simulink subsystem "Plant_and_Environment_Model"  (R2020a)
settings: Solver=VariableStepAuto  StartTime=0.0  StopTime=10.0  RelTol=1e-3
values from neighbouring files (symbols this model uses):
  a_rad = deg2rad(a)    [plant_init.m]
  AF = [0.12, 0.22, 0.292]    [plant_init.m]
  l1 = [ sin(a14),-cos(a14), 0,         (D14(3)-RG(3)+PZ(1)*dz)*cos(a14),         (D14(3)-RG(3)+PZ(1)*dz)*sin(a14),         -hypot( D14(1)-RG(1), D14(2)-RG(2))]    [GetAuvSimAndJacobian.m]    (also in plant_init.m = [(D14(3)-RB(3)+PZ(1)*dz),     (D14(3)-RB(3)+PZ(1)*dz),     -)
  l2 = [ sin(a14), cos(a14), 0,          -(D14(3)-RG(3)+PZ(2)*dz)*cos(a14),          (D14(3)-RG(3)+PZ(2)*dz)*sin(a14),          -hypot( D14(1)+RG(1), D14(2)-RG(2))]    [GetAuvSimAndJacobian.m]    (also in plant_init.m = [-(D14(3)-RB(3)+PZ(2)*dz),      (D14(3)-RB(3)+PZ(2)*dz),    )
  l3 = [ sin(a14),-cos(a14), 0,         (D14(3)-RG(3)+PZ(3)*dz)*cos(a14),          (D14(3)-RG(3)+PZ(3)*dz)*sin(a14),          hypot(D14(1)+RG(1), D14(2)+RG(2))]    [GetAuvSimAndJacobian.m]    (also in plant_init.m = [(D14(3)-RB(3)+PZ(3)*dz),      (D14(3)-RB(3)+PZ(3)*dz),     )
  l4 = [ sin(a14), cos(a14), 0,         -(D14(3)-RG(3)+PZ(4)*dz)*cos(a14),          (D14(3)-RG(3)+PZ(4)*dz)*sin(a14),          hypot(D14(1)-RG(1), D14(2)+RG(2))]    [GetAuvSimAndJacobian.m]    (also in plant_init.m = [-(D14(3)-RB(3)+PZ(4)*dz),      (D14(3)-RB(3)+PZ(4)*dz),    )
  l5 = [0, 0, 1, (D58(2)-RG(2)+PZ(1)*dz),          -(D58(1)-RG(1)+PZ(1)*dz), 0]    [GetAuvSimAndJacobian.m]    (also in plant_init.m = [(D58(2)-RB(2)+PZ(1)*dz),      -(D58(1)-RB(1)+PZ(1)*dz), 0])
  l6 = [0, 0,-1,-(D58(2)-RG(2)+PZ(2)*dz),           -(D58(1)+RG(1)+PZ(2)*dz), 0]    [GetAuvSimAndJacobian.m]    (also in plant_init.m = [-(D58(2)-RB(2)+PZ(2)*dz),       -(D58(1)+RB(1)+PZ(2)*dz), 0)
  l7 = [0, 0, 1,-(D58(2)+RG(2)+PZ(3)*dz),         (D58(1)+RG(1)+PZ(3)*dz), 0]    [GetAuvSimAndJacobian.m]    (also in plant_init.m = [-(D58(2)+RB(2)+PZ(3)*dz),     (D58(1)+RB(1)+PZ(3)*dz), 0])
  l8 = [0, 0,-1, (D58(2)+RG(2)+PZ(4)*dz),          (D58(1)-RG(1)+PZ(2)*dz), 0]    [GetAuvSimAndJacobian.m]    (also in plant_init.m = [(D58(2)+RB(2)+PZ(4)*dz),      (D58(1)-RB(1)+PZ(2)*dz), 0])
  mass = cf.mass    [main_adaptive_mpc.m]    (also in plant_init.m = 33.95)
  N = [-39.9215617836 -39.7361560536 -39.4691718024 -38.8907059248 -38.267742672 -37.9562610456 -37.5112872936 -37.2888004176 -36.7993292904 -36.4433502888 -35.8648844112 -35.1974237832 ... (201 elements, 201x1)]    [matlab.mat]    (also in plant_init.m = T200Spec16V{:,6})
  PWM = [1100 1104 1108 1112 1116 1120 1124 1128 1132 1136 1140 1144 ... (201 elements, 201x1)]    [matlab.mat]    (also in plant_init.m = T200Spec16V{:,1})
  RB = [ 0.001,      -0.003,       0.027]    [plant_init.m]
  RG = [ 0.001,      -0.003,       0.027]    [plant_init.m]
  rho = 998    [plant_init.m]
  volume = 0.027    [plant_init.m]
libraries: sharedtransform x11, vrlib x9, shared6dof x1, aerolibasang x1
(part 2 of 2)

== system Plant_and_Environment_Model/Propulsion Forces & Moments/Force and moments due to Thrust/Thrust to Propulsion /Moment computation/Moment Moteur 4 ==
  Thrust : Inport
  Constant : Constant  Value=[a;b;c]
  Cross Product : vrlib/Utilities/Cross Product
  Moment : Outport  VectorParamsAs1DForOutWhenUnconnected=off
  wires:
  Cross Product/1 -> Moment/1
  Thrust/1 -> Cross Product/2
  Constant/1 -> Cross Product/1

== system Plant_and_Environment_Model/Propulsion Forces & Moments/Force and moments due to Thrust/Thrust to Propulsion /Moment computation/Moment Moteur 5 ==
  Thrust : Inport
  Constant : Constant  Value=[a;b;c]
  Cross Product : vrlib/Utilities/Cross Product
  Moment : Outport  VectorParamsAs1DForOutWhenUnconnected=off
  wires:
  Constant/1 -> Cross Product/1
  Thrust/1 -> Cross Product/2
  Cross Product/1 -> Moment/1

== system Plant_and_Environment_Model/Propulsion Forces & Moments/Force and moments due to Thrust/Thrust to Propulsion /Moment computation/Moment Moteur 6 ==
  Thrust : Inport
  Constant : Constant  Value=[a;b;c]
  Cross Product : vrlib/Utilities/Cross Product
  Moment : Outport  VectorParamsAs1DForOutWhenUnconnected=off
  wires:
  Constant/1 -> Cross Product/1
  Thrust/1 -> Cross Product/2
  Cross Product/1 -> Moment/1

== system Plant_and_Environment_Model/Propulsion Forces & Moments/Force and moments due to Thrust/Thrust to Propulsion /Moment computation/Moment Moteur 7 ==
  Thrust : Inport
  Constant : Constant  Value=[a;b;c]
  Cross Product : vrlib/Utilities/Cross Product
  Moment : Outport  VectorParamsAs1DForOutWhenUnconnected=off
  wires:
  Constant/1 -> Cross Product/1
  Thrust/1 -> Cross Product/2
  Cross Product/1 -> Moment/1

== system Plant_and_Environment_Model/Propulsion Forces & Moments/Force and moments due to Thrust/Thrust to Propulsion /Moment computation/Moment Moteur 8 ==
  Thrust : Inport
  Constant : Constant  Value=[a;b;c]
  Cross Product : vrlib/Utilities/Cross Product
  Moment : Outport  VectorParamsAs1DForOutWhenUnconnected=off
  wires:
  Constant/1 -> Cross Product/1
  Thrust/1 -> Cross Product/2
  Cross Product/1 -> Moment/1

== matlab function Plant_and_Environment_Model/Environmental Forces & Moments/Hydrodynamic Forces/Hydrodynamic Forces - Accurate/Force Exerted due to Lift (Body Axis)/MATLAB Function ==
  data: u input; y output
function y = fcn(u)
if u>pi/2
    u = u-pi;
elseif u < -pi/2
    u = u + pi;
end

y = 1 * (u) + 0;

== matlab function Plant_and_Environment_Model/Propulsion Forces & Moments/Input commands to Thrust/PWM Signals to Thrust /MATLAB Function ==
  data: u input; y output
function y = Normalize(u)
y = (u-1500)*150/400;

== matlab function Plant_and_Environment_Model/Propulsion Forces & Moments/Input commands to Thrust/PWM Signals to Thrust /MATLAB Function1 ==
  data: u input; y output
function y = Normalize(u)
y = (u-1500)*150/400;

== matlab function Plant_and_Environment_Model/Propulsion Forces & Moments/Input commands to Thrust/PWM Signals to Thrust /MATLAB Function2 ==
  data: u input; y output
function y = Normalize(u)
y = (u-1500)*150/400;

== matlab function Plant_and_Environment_Model/Propulsion Forces & Moments/Input commands to Thrust/PWM Signals to Thrust /MATLAB Function3 ==
  data: u input; y output
function y = Normalize(u)
y = (u-1500)*150/400;

== matlab function Plant_and_Environment_Model/Propulsion Forces & Moments/Input commands to Thrust/PWM Signals to Thrust /MATLAB Function4 ==
  data: u input; y output
function y = Normalize(u)
y = (u-1500)*150/400;

== matlab function Plant_and_Environment_Model/Dynamics solver/Post-Processing/MATLAB Function ==
  data: Position input; srf_in input
function Visualize(Position, srf_in)

    coder.extrinsic('setax'); 
    setax(Position, srf_in);  

end

== matlab function Plant_and_Environment_Model/Propulsion Forces & Moments/Input commands to Thrust/PWM Signals to Thrust /MATLAB Function5 ==
  data: u input; y output
function y = Normalize(u)
y = (u-1500)*150/400;

== matlab function Plant_and_Environment_Model/Propulsion Forces & Moments/Input commands to Thrust/PWM Signals to Thrust /MATLAB Function6 ==
  data: u input; y output
function y = Normalize(u)
y = (u-1500)*150/400;

== matlab function Plant_and_Environment_Model/Propulsion Forces & Moments/Input commands to Thrust/PWM Signals to Thrust /MATLAB Function7 ==
  data: u input; y output
function y = Normalize(u)
y = (u-1500)*150/400;

== matlab function Plant_and_Environment_Model/Environmental Forces & Moments/Hydrodynamic Forces/Hydrodynamic Forces - Accurate/Force Exerted due to Drag (Body Axis)/MATLAB Function ==
  data: u input; C_D output
function C_D = Calculate_Drag_Coeff(u)
if u>pi/2
    u = u-pi;
elseif u < -pi/2
    u = u + pi;
end
C_D = 5.25*(u.^2) - 0.315 * (u) + 0.732;
